simulink model "LAB_07_SIM_GG_SRP"  (R2022b)
settings: Solver=ode8  StartTime=0.0  StopTime=10000  FixedStep=0.05  RelTol=1e-3
values from neighbouring files (symbols this model uses):
  a = 16371e+3    (= 16371000)    [lab_07_MAT.m]
  A0 = diag([1 1 1])    [LAB_04_17_OCT_MAT_KIN.m]    (also in LAB_05_24_OCT_MAT_KIN_COSDIR.m; LAB_06.m = A_target_fun(0); core_attitude_test.m = eye(3,3); lab_07_MAT.m)
  A_B1 = 2e-2    (= 0.02)    [lab_07_MAT.m]
  A_B2 = 6e-2    (= 0.06)    [lab_07_MAT.m]
  A_B3 = 2e-2    (= 0.02)    [lab_07_MAT.m]
  A_B4 = 6e-2    (= 0.06)    [lab_07_MAT.m]
  A_B5 = 3e-2    (= 0.03)    [lab_07_MAT.m]
  A_B6 = 3e-2    (= 0.03)    [lab_07_MAT.m]
  A_P1 = 12e-2    (= 0.12)    [lab_07_MAT.m]
  A_P2 = 12e-2    (= 0.12)    [lab_07_MAT.m]
  A_P3 = 12e-2    (= 0.12)    [lab_07_MAT.m]
  A_P4 = 12e-2    (= 0.12)    [lab_07_MAT.m]
  ang = deg2rad(11.5)    [lab_07_MAT.m]
  e = 0    [lab_07_MAT.m]
  G = 6.67430e-11    (= 6.6743e-11)    [LAB_06.m]    (also in lab_07_MAT.m)
  g_1_0 = -29404.8    [lab_07_MAT.m]
  g_1_1 = -1450.9    [lab_07_MAT.m]
  h_1_1 = 4652.5    [lab_07_MAT.m]
  i = char('pippo')    [LAB_01_19_SEPT.m]    (also in lab_07_MAT.m = 0.1)
  I = [Ix 0 0 ... (first row only)    [LAB_03_3_OCT_MAT_EUL_2_VERIFICATION.m]    (also in LAB_03_3_OCT_MAT_EUL_DOUBLESPIN.m = diag([Ix, Iy, Iz]); LAB_03_3_OCT_MAT_EUL_SPINAXIS.m = diag([Ix, Iy, Iz]); LAB_03_3_OCT_MAT_EUL_VECT.m; LAB_04_17_OCT_MAT_KIN.m)
  j_B = [0.01; 0.05; 0.01]    [lab_07_MAT.m]
  Mt = 5.972e+24    [LAB_06.m]    (also in lab_07_MAT.m)
  N_B1 = [1,0,0]'    [lab_07_MAT.m]
  N_B2 = [0,1,0]'    [lab_07_MAT.m]
  N_B3 = [-1,0,0]'    [lab_07_MAT.m]
  N_B4 = [0,-1,0]'    [lab_07_MAT.m]
  N_B5 = [0,0,1]'    [lab_07_MAT.m]
  N_B6 = [0,0,-1]    [lab_07_MAT.m]
  N_P1 = [0,0,1]    [lab_07_MAT.m]
  N_P2 = [0,0,-1]    [lab_07_MAT.m]
  N_P3 = [0,0,1]    [lab_07_MAT.m]
  N_P4 = [0,0,-1]    [lab_07_MAT.m]
  n_rot = 0.0012    [lab_07_MAT.m]
  n_sun = 2*pi/T    (= 1.99238499086e-07)    [lab_07_MAT.m]
  om_0 = [om_x0, om_y0, om_z0]    [LAB_03_3_OCT_MAT_EUL.m]    (also in LAB_03_3_OCT_MAT_EUL_2_VERIFICATION.m = [om_x0; om_y0; om_z0]; LAB_03_3_OCT_MAT_EUL_DOUBLESPIN.m = [om_x0; om_y0; om_z0]; LAB_03_3_OCT_MAT_EUL_SPINAXIS.m = [om_x0; om_y0; om_z0]; LAB_03_3_OCT_MAT_EUL_VECT.m = [om_x0; om_y0; om_z0])
  om_target = [0; 0; n]    [LAB_06.m]    (also in lab_07_MAT.m)
  P = [Px, Py, Pz]    [LAB_03_3_OCT_MAT_EUL_VECT.m]    (also in lab_07_MAT.m = 4.52666666667e-06)
  R = 6.371e+6 + H    (= 6381000)    [LAB_06.m]    (also in lab_07_MAT.m = 6378000)
  r_B1 = 1e-2*[15,0,0]    [lab_07_MAT.m]
  r_B2 = 1e-2*[0,5,0]    [lab_07_MAT.m]
  r_B3 = 1e-2*[-15,0,0]    [lab_07_MAT.m]
  r_B4 = 1e-2*[0,-5,0]    [lab_07_MAT.m]
  r_B5 = 1e-2*[0,0,10]    [lab_07_MAT.m]
  r_B6 = 1e-2*[0,0,-10]    [lab_07_MAT.m]
  r_P1 = 1e-2*[0,20,10]    [lab_07_MAT.m]
  r_P2 = 1e-2*[0,20,10]    [lab_07_MAT.m]
  r_P3 = 1e-2*[0,-20,10]    [lab_07_MAT.m]
  r_P4 = 1e-2*[0,-20,10]    [lab_07_MAT.m]
  r_sun = 149597870000    [lab_07_MAT.m]
  rho_d = 0.1    [lab_07_MAT.m]
  rho_sB = 0.5    [lab_07_MAT.m]
  rho_sP = 0.5    [lab_07_MAT.m]
  rot_E = 7.29e-5    (= 7.29e-05)    [lab_07_MAT.m]
  theta_0 = 3/2 * pi    (= 4.71238898038)    [lab_07_MAT.m]
libraries: matrix_library x17, sharedutil x3, vrlib x1
(part 2 of 2)

== system LAB_07_SIM_GG_SRP/Dynamics gg and srp/validation/norm ==
  Input : Inport
  Demux : Demux  Outputs=3
  Sqrt : Sqrt
  Square : Math  Operator=square
  Square1 : Math  Operator=square
  Square2 : Math  Operator=square
  Sum : Sum  Inputs=+++
  Output : Outport
  wires:
  Square/1 -> Sum/1
  Square1/1 -> Sum/2
  Square2/1 -> Sum/3
  Sum/1 -> Sqrt/1
  Input/1 -> Demux/1
  Sqrt/1 -> Output/1
  Demux/1 -> Square/1
  Demux/2 -> Square1/1
  Demux/3 -> Square2/1

== system LAB_07_SIM_GG_SRP/Magnetic field and torque/m/norm ==
  Input : Inport
  Demux : Demux  Outputs=3
  Sqrt : Sqrt
  Square : Math  Operator=square
  Square1 : Math  Operator=square
  Square2 : Math  Operator=square
  Sum : Sum  Inputs=+++
  Output : Outport
  wires:
  Square/1 -> Sum/1
  Square1/1 -> Sum/2
  Square2/1 -> Sum/3
  Sum/1 -> Sqrt/1
  Input/1 -> Demux/1
  Sqrt/1 -> Output/1
  Demux/1 -> Square/1
  Demux/2 -> Square1/1
  Demux/3 -> Square2/1

== system LAB_07_SIM_GG_SRP/Subsystem/DCM/Determinant Chech fo Validation ==
  DCM : Inport
  Determinant of 3x3 Matrix : sharedutil/Determinant of 3x3 Matrix  aMode=aMode
      settings: LibrarySourceBlock=|
      | aerolibutil/Determinant of
      | 3x3 Matrix
  MATLAB Function : MATLAB Function  TreatAsAtomicUnit=on
  determinant : Scope
  perpendicularity : Scope
  wires:
  Determinant of 3x3 Matrix/1 -> determinant/1
  DCM/1 -> MATLAB Function/1(DCM), Determinant of 3x3 Matrix/1
  MATLAB Function/1(perpendicularity_flag) -> perpendicularity/1

== system LAB_07_SIM_GG_SRP/Subsystem/DCM/Subsystem ==
  A1 : Inport
  Gain : Gain  Gain=1.5
  Gain1 : Gain  Gain=-0.5
  Product : Product  Inputs=3  Multiplication=Matrix(*)
  Sum1 : Sum
  Transpose1 : Math  Operator=transpose
  A_orthonormalized1 : Outport
  wires:
  A1/1 -> Product/1, Transpose1/1, Product/3, Gain/1
  Gain/1 -> Sum1/2
  Sum1/1 -> A_orthonormalized1/1
  Gain1/1 -> Sum1/1
  Product/1 -> Gain1/1
  Transpose1/1 -> Product/2

== system LAB_07_SIM_GG_SRP/Subsystem/DCM/matrix of omega cross prod ==
  om : Inport
  Constant1 : Constant  Value=0
  Constant2 : Constant  Value=0
  Constant3 : Constant  Value=0
  Demux : Demux  Outputs=3
  Gain : Gain  Gain=-1
  Gain1 : Gain  Gain=-1
  Gain2 : Gain  Gain=-1
  Matrix Concatenate : Concatenate  NumInputs=3  Mode=Multidimensional array
  Mux : Mux  Inputs=3
  Mux1 : Mux  Inputs=3
  Mux2 : Mux  Inputs=3
  Scope : Scope
  Transpose : Math  Operator=transpose
  Transpose1 : Math  Operator=transpose
  Transpose2 : Math  Operator=transpose
  Out1 : Outport
  wires:
  Matrix Concatenate/1 -> Scope/1, Out1/1
  Demux/1 -> Gain1/1, Mux2/2
  Mux1/1 -> Transpose1/1
  Constant3/1 -> Mux2/3
  Gain/1 -> Mux/2
  Gain2/1 -> Mux2/1
  Constant1/1 -> Mux/1
  Demux/3 -> Gain/1, Mux1/1
  Demux/2 -> Mux/3, Gain2/1
  Mux/1 -> Transpose/1
  Gain1/1 -> Mux1/3
  Mux2/1 -> Transpose2/1
  Constant2/1 -> Mux1/2
  om/1 -> Demux/1
  Transpose/1 -> Matrix Concatenate/1
  Transpose1/1 -> Matrix Concatenate/2
  Transpose2/1 -> Matrix Concatenate/3

== matlab function LAB_07_SIM_GG_SRP/DCM/Determinant Chech fo Validation/MATLAB Function ==
  data: DCM input; perpendicularity_flag output
 function perpendicularity_flag = fcn(DCM)


perpendicularity_flag =zeros(3,1);

    x   = DCM(1,:);
    y   = DCM(2,:);
    z   = DCM(3,:);

    perpendicularity_flag(1)=dot(x,y);
    perpendicularity_flag(2)=dot(x,z);
    perpendicularity_flag(3)=dot(z,y);

end

== matlab function LAB_07_SIM_GG_SRP/Subsystem/Check_Orthogonality_V/MATLAB Function2 ==
  data: S input; perpp_flag output
function perpp_flag = fcn(S)


perpp_flag =zeros(3,1);

    x   = S(:,1);
    y   = S(:,2);
    z   = S(:,3);

    perpp_flag(1)=dot(x,y);
    perpp_flag(2)=dot(x,z);
    perpp_flag(3)=dot(z,y);

end

== matlab function LAB_07_SIM_GG_SRP/Subsystem/DCM/Determinant Chech fo Validation/MATLAB Function ==
  data: DCM input; perpendicularity_flag output
 function perpendicularity_flag = fcn(DCM)


perpendicularity_flag =zeros(3,1);

    x   = DCM(1,:);
    y   = DCM(2,:);
    z   = DCM(3,:);

    perpendicularity_flag(1)=dot(x,y);
    perpendicularity_flag(2)=dot(x,z);
    perpendicularity_flag(3)=dot(z,y);

end

== matlab function LAB_07_SIM_GG_SRP/Subsystem/Check_Orthogonality_S/MATLAB Function1 ==
  data: S input; perp_flag output
 function perp_flag = fcn(S)


perp_flag =zeros(3,1);

    x   = S(:,1);
    y   = S(:,2);
    z   = S(:,3);

    perp_flag(1)=dot(x,y);
    perp_flag(2)=dot(x,z);
    perp_flag(3)=dot(z,y);

end
